simulink model "c00006M_harness"  (R2018a)
settings: Solver=FixedStepAuto  StartTime=0.0  StopTime=300  FixedStep=0.1  RelTol=1e-3
undefined symbols (not defined in the file): A1, hmax, PriorityTank, R1, R2, sigbuilder_block, TempThreshold
(part 15 of 66)

== system c00006M_harness/M205/Tank3 ==
  CT3 : Inport
  F3 : Inport  Port=2
  E3 : Inport  Port=3
  MR3 : Inport  Port=4
  T3 : Inport  Port=5
  EB3 : Inport  Port=6
  LL2 : Inport  Port=7
  Control : Subsystem
  Logical Operator : Logic  AllPortsSameDT=off  OutDataTypeStr=boolean
  MasterTankControl : Subsystem
  Memory : Memory
  Memory2 : Memory
  TankModel : Subsystem
  LL3 : Outport
  wires:
  TankModel/1(LiquidLevel) -> Memory/1, LL3/1
  Control/1(LiquidIn) -> Logical Operator/1
  Control/2(LiquidOut) -> TankModel/2(LiquidOut)
  Memory/1 -> MasterTankControl/2(LiquidTank3), Control/8(LiquidLevel)
  MR3/1 -> Control/3(ManualReference)
  CT3/1 -> Control/2(StartMaintenance), Control/1(ControlType)
  F3/1 -> Control/4(Fill)
  E3/1 -> Control/5(Empty)
  LL2/1 -> Memory2/1
  Memory2/1 -> MasterTankControl/1(LiquidTank2)
  EB3/1 -> Control/6(EmergencyButton)
  MasterTankControl/1(AllowTheTankFilling) -> Logical Operator/2
  Logical Operator/1 -> TankModel/1(LiquidIn)
  T3/1 -> Control/7(Temperature)

== system c00006M_harness/M206/Tank2 ==
  CT2 : Inport
  F2 : Inport  Port=2
  E2 : Inport  Port=3
  MR2 : Inport  Port=4
  T2 : Inport  Port=5
  EB2 : Inport  Port=6
  LL3 : Inport  Port=7
  Control : Subsystem
  Logical Operator : Logic  AllPortsSameDT=off  OutDataTypeStr=boolean
  MasterTankControl : Subsystem
  Memory : Memory
  Memory2 : Memory
  TankModel : Subsystem
  LL2 : Outport
  wires:
  TankModel/1(LiquidLevel) -> Memory/1, LL2/1
  Control/1(LiquidIn) -> Logical Operator/1
  Control/2(LiquidOut) -> TankModel/2(LiquidOut)
  Memory/1 -> Control/8(LiquidLevel), MasterTankControl/1(LiquidTank2)
  MR2/1 -> Control/3(ManualReference)
  CT2/1 -> Control/2(StartMaintenance), Control/1(ControlType)
  F2/1 -> Control/4(Fill)
  E2/1 -> Control/5(Empty)
  LL3/1 -> Memory2/1
  Memory2/1 -> MasterTankControl/2(LiquidTank3)
  EB2/1 -> Control/6(EmergencyButton)
  MasterTankControl/1(AllowTheTankFilling) -> Logical Operator/2
  Logical Operator/1 -> TankModel/1(LiquidIn)
  T2/1 -> Control/7(Temperature)

== system c00006M_harness/M206/Tank3 ==
  CT3 : Inport
  F3 : Inport  Port=2
  E3 : Inport  Port=3
  MR3 : Inport  Port=4
  T3 : Inport  Port=5
  EB3 : Inport  Port=6
  LL2 : Inport  Port=7
  Control : Subsystem
  Logical Operator : Logic  AllPortsSameDT=off  OutDataTypeStr=boolean
  MasterTankControl : Subsystem
  Memory : Memory
  Memory2 : Memory
  TankModel : Subsystem
  LL3 : Outport
  wires:
  TankModel/1(LiquidLevel) -> Memory/1, LL3/1
  Control/1(LiquidIn) -> Logical Operator/1
  Control/2(LiquidOut) -> TankModel/2(LiquidOut)
  Memory/1 -> MasterTankControl/2(LiquidTank3), Control/8(LiquidLevel)
  MR3/1 -> Control/3(ManualReference)
  CT3/1 -> Control/2(StartMaintenance), Control/1(ControlType)
  F3/1 -> Control/4(Fill)
  E3/1 -> Control/5(Empty)
  LL2/1 -> Memory2/1
  Memory2/1 -> MasterTankControl/1(LiquidTank2)
  EB3/1 -> Control/6(EmergencyButton)
  MasterTankControl/1(AllowTheTankFilling) -> Logical Operator/2
  Logical Operator/1 -> TankModel/1(LiquidIn)
  T3/1 -> Control/7(Temperature)

== system c00006M_harness/M207/Tank2 ==
  CT2 : Inport
  F2 : Inport  Port=2
  E2 : Inport  Port=3
  MR2 : Inport  Port=4
  T2 : Inport  Port=5
  EB2 : Inport  Port=6
  LL3 : Inport  Port=7
  Control : Subsystem
  Logical Operator : Logic  AllPortsSameDT=off  OutDataTypeStr=boolean
  MasterTankControl : Subsystem
  Memory : Memory
  Memory2 : Memory
  TankModel : Subsystem
  LL2 : Outport
  wires:
  TankModel/1(LiquidLevel) -> Memory/1, LL2/1
  Control/1(LiquidIn) -> Logical Operator/1
  Control/2(LiquidOut) -> TankModel/2(LiquidOut)
  Memory/1 -> Control/8(LiquidLevel), MasterTankControl/1(LiquidTank2)
  MR2/1 -> Control/3(ManualReference)
  CT2/1 -> Control/2(StartMaintenance), Control/1(ControlType)
  F2/1 -> Control/4(Fill)
  E2/1 -> Control/5(Empty)
  LL3/1 -> Memory2/1
  Memory2/1 -> MasterTankControl/2(LiquidTank3)
  EB2/1 -> Control/6(EmergencyButton)
  MasterTankControl/1(AllowTheTankFilling) -> Logical Operator/2
  Logical Operator/1 -> TankModel/1(LiquidIn)
  T2/1 -> Control/7(Temperature)

== system c00006M_harness/M207/Tank3 ==
  CT3 : Inport
  F3 : Inport  Port=2
  E3 : Inport  Port=3
  MR3 : Inport  Port=4
  T3 : Inport  Port=5
  EB3 : Inport  Port=6
  LL2 : Inport  Port=7
  Control : Subsystem
  Logical Operator : Logic  AllPortsSameDT=off  OutDataTypeStr=boolean
  MasterTankControl : Subsystem
  Memory : Memory
  Memory2 : Memory
  TankModel : Subsystem
  LL3 : Outport
  wires:
  TankModel/1(LiquidLevel) -> Memory/1, LL3/1
  Control/1(LiquidIn) -> Logical Operator/1
  Control/2(LiquidOut) -> TankModel/2(LiquidOut)
  Memory/1 -> MasterTankControl/2(LiquidTank3), Control/8(LiquidLevel)
  MR3/1 -> Control/3(ManualReference)
  CT3/1 -> Control/2(StartMaintenance), Control/1(ControlType)
  F3/1 -> Control/4(Fill)
  E3/1 -> Control/5(Empty)
  LL2/1 -> Memory2/1
  Memory2/1 -> MasterTankControl/1(LiquidTank2)
  EB3/1 -> Control/6(EmergencyButton)
  MasterTankControl/1(AllowTheTankFilling) -> Logical Operator/2
  Logical Operator/1 -> TankModel/1(LiquidIn)
  T3/1 -> Control/7(Temperature)

== system c00006M_harness/M208/Tank2 ==
  CT2 : Inport
  F2 : Inport  Port=2
  E2 : Inport  Port=3
  MR2 : Inport  Port=4
  T2 : Inport  Port=5
  EB2 : Inport  Port=6
  LL3 : Inport  Port=7
  Control : Subsystem
  Logical Operator : Logic  AllPortsSameDT=off  OutDataTypeStr=boolean
  MasterTankControl : Subsystem
  Memory : Memory
  Memory2 : Memory
  TankModel : Subsystem
  LL2 : Outport
  wires:
  TankModel/1(LiquidLevel) -> Memory/1, LL2/1
  Control/1(LiquidIn) -> Logical Operator/1
  Control/2(LiquidOut) -> TankModel/2(LiquidOut)
  Memory/1 -> Control/8(LiquidLevel), MasterTankControl/1(LiquidTank2)
  MR2/1 -> Control/3(ManualReference)
  CT2/1 -> Control/2(StartMaintenance), Control/1(ControlType)
  F2/1 -> Control/4(Fill)
  E2/1 -> Control/5(Empty)
  LL3/1 -> Memory2/1
  Memory2/1 -> MasterTankControl/2(LiquidTank3)
  EB2/1 -> Control/6(EmergencyButton)
  MasterTankControl/1(AllowTheTankFilling) -> Logical Operator/2
  Logical Operator/1 -> TankModel/1(LiquidIn)
  T2/1 -> Control/7(Temperature)

== system c00006M_harness/M208/Tank3 ==
  CT3 : Inport
  F3 : Inport  Port=2
  E3 : Inport  Port=3
  MR3 : Inport  Port=4
  T3 : Inport  Port=5
  EB3 : Inport  Port=6
  LL2 : Inport  Port=7
  Control : Subsystem
  Logical Operator : Logic  AllPortsSameDT=off  OutDataTypeStr=boolean
  MasterTankControl : Subsystem
  Memory : Memory
  Memory2 : Memory
  TankModel : Subsystem
  LL3 : Outport
  wires:
  TankModel/1(LiquidLevel) -> Memory/1, LL3/1
  Control/1(LiquidIn) -> Logical Operator/1
  Control/2(LiquidOut) -> TankModel/2(LiquidOut)
  Memory/1 -> MasterTankControl/2(LiquidTank3), Control/8(LiquidLevel)
  MR3/1 -> Control/3(ManualReference)
  CT3/1 -> Control/2(StartMaintenance), Control/1(ControlType)
  F3/1 -> Control/4(Fill)
  E3/1 -> Control/5(Empty)
  LL2/1 -> Memory2/1
  Memory2/1 -> MasterTankControl/1(LiquidTank2)
  EB3/1 -> Control/6(EmergencyButton)
  MasterTankControl/1(AllowTheTankFilling) -> Logical Operator/2
  Logical Operator/1 -> TankModel/1(LiquidIn)
  T3/1 -> Control/7(Temperature)

== system c00006M_harness/M209/Tank2 ==
  CT2 : Inport
  F2 : Inport  Port=2
  E2 : Inport  Port=3
  MR2 : Inport  Port=4
  T2 : Inport  Port=5
  EB2 : Inport  Port=6
  LL3 : Inport  Port=7
  Control : Subsystem
  Logical Operator : Logic  AllPortsSameDT=off  OutDataTypeStr=boolean
  MasterTankControl : Subsystem
  Memory : Memory
  Memory2 : Memory
  TankModel : Subsystem
  LL2 : Outport
  wires:
  TankModel/1(LiquidLevel) -> Memory/1, LL2/1
  Control/1(LiquidIn) -> Logical Operator/1
  Control/2(LiquidOut) -> TankModel/2(LiquidOut)
  Memory/1 -> Control/8(LiquidLevel), MasterTankControl/1(LiquidTank2)
  MR2/1 -> Control/3(ManualReference)
  CT2/1 -> Control/2(StartMaintenance), Control/1(ControlType)
  F2/1 -> Control/4(Fill)
  E2/1 -> Control/5(Empty)
  LL3/1 -> Memory2/1
  Memory2/1 -> MasterTankControl/2(LiquidTank3)
  EB2/1 -> Control/6(EmergencyButton)
  MasterTankControl/1(AllowTheTankFilling) -> Logical Operator/2
  Logical Operator/1 -> TankModel/1(LiquidIn)
  T2/1 -> Control/7(Temperature)

== system c00006M_harness/M209/Tank3 ==
  CT3 : Inport
  F3 : Inport  Port=2
  E3 : Inport  Port=3
  MR3 : Inport  Port=4
  T3 : Inport  Port=5
  EB3 : Inport  Port=6
  LL2 : Inport  Port=7
  Control : Subsystem
  Logical Operator : Logic  AllPortsSameDT=off  OutDataTypeStr=boolean
  MasterTankControl : Subsystem
  Memory : Memory
  Memory2 : Memory
  TankModel : Subsystem
  LL3 : Outport
  wires:
  TankModel/1(LiquidLevel) -> Memory/1, LL3/1
  Control/1(LiquidIn) -> Logical Operator/1
  Control/2(LiquidOut) -> TankModel/2(LiquidOut)
  Memory/1 -> MasterTankControl/2(LiquidTank3), Control/8(LiquidLevel)
  MR3/1 -> Control/3(ManualReference)
  CT3/1 -> Control/2(StartMaintenance), Control/1(ControlType)
  F3/1 -> Control/4(Fill)
  E3/1 -> Control/5(Empty)
  LL2/1 -> Memory2/1
  Memory2/1 -> MasterTankControl/1(LiquidTank2)
  EB3/1 -> Control/6(EmergencyButton)
  MasterTankControl/1(AllowTheTankFilling) -> Logical Operator/2
  Logical Operator/1 -> TankModel/1(LiquidIn)
  T3/1 -> Control/7(Temperature)

== system c00006M_harness/M210/Tank2 ==
  CT2 : Inport
  F2 : Inport  Port=2
  E2 : Inport  Port=3
  MR2 : Inport  Port=4
  T2 : Inport  Port=5
  EB2 : Inport  Port=6
  LL3 : Inport  Port=7
  Control : Subsystem
  Logical Operator : Logic  AllPortsSameDT=off  OutDataTypeStr=boolean
  MasterTankControl : Subsystem
  Memory : Memory
  Memory2 : Memory
  TankModel : Subsystem
  LL2 : Outport
  wires:
  TankModel/1(LiquidLevel) -> Memory/1, LL2/1
  Control/1(LiquidIn) -> Logical Operator/1
  Control/2(LiquidOut) -> TankModel/2(LiquidOut)
  Memory/1 -> Control/8(LiquidLevel), MasterTankControl/1(LiquidTank2)
  MR2/1 -> Control/3(ManualReference)
  CT2/1 -> Control/2(StartMaintenance), Control/1(ControlType)
  F2/1 -> Control/4(Fill)
  E2/1 -> Control/5(Empty)
  LL3/1 -> Memory2/1
  Memory2/1 -> MasterTankControl/2(LiquidTank3)
  EB2/1 -> Control/6(EmergencyButton)
  MasterTankControl/1(AllowTheTankFilling) -> Logical Operator/2
  Logical Operator/1 -> TankModel/1(LiquidIn)
  T2/1 -> Control/7(Temperature)

== system c00006M_harness/M210/Tank3 ==
  CT3 : Inport
  F3 : Inport  Port=2
  E3 : Inport  Port=3
  MR3 : Inport  Port=4
  T3 : Inport  Port=5
  EB3 : Inport  Port=6
  LL2 : Inport  Port=7
  Control : Subsystem
  Logical Operator : Logic  AllPortsSameDT=off  OutDataTypeStr=boolean
  MasterTankControl : Subsystem
  Memory : Memory
  Memory2 : Memory
  TankModel : Subsystem
  LL3 : Outport
  wires:
  TankModel/1(LiquidLevel) -> Memory/1, LL3/1
  Control/1(LiquidIn) -> Logical Operator/1
  Control/2(LiquidOut) -> TankModel/2(LiquidOut)
  Memory/1 -> MasterTankControl/2(LiquidTank3), Control/8(LiquidLevel)
  MR3/1 -> Control/3(ManualReference)
  CT3/1 -> Control/2(StartMaintenance), Control/1(ControlType)
  F3/1 -> Control/4(Fill)
  E3/1 -> Control/5(Empty)
  LL2/1 -> Memory2/1
  Memory2/1 -> MasterTankControl/1(LiquidTank2)
  EB3/1 -> Control/6(EmergencyButton)
  MasterTankControl/1(AllowTheTankFilling) -> Logical Operator/2
  Logical Operator/1 -> TankModel/1(LiquidIn)
  T3/1 -> Control/7(Temperature)

== system c00006M_harness/M211/Tank2 ==
  CT2 : Inport
  F2 : Inport  Port=2
  E2 : Inport  Port=3
  MR2 : Inport  Port=4
  T2 : Inport  Port=5
  EB2 : Inport  Port=6
  LL3 : Inport  Port=7
  Control : Subsystem
  Logical Operator : Logic  AllPortsSameDT=off  OutDataTypeStr=boolean
  MasterTankControl : Subsystem
  Memory : Memory
  Memory2 : Memory
  TankModel : Subsystem
  LL2 : Outport
  wires:
  TankModel/1(LiquidLevel) -> Memory/1, LL2/1
  Control/1(LiquidIn) -> Logical Operator/1
  Control/2(LiquidOut) -> TankModel/2(LiquidOut)
  Memory/1 -> Control/8(LiquidLevel), MasterTankControl/1(LiquidTank2)
  MR2/1 -> Control/3(ManualReference)
  CT2/1 -> Control/2(StartMaintenance), Control/1(ControlType)
  F2/1 -> Control/4(Fill)
  E2/1 -> Control/5(Empty)
  LL3/1 -> Memory2/1
  Memory2/1 -> MasterTankControl/2(LiquidTank3)
  EB2/1 -> Control/6(EmergencyButton)
  MasterTankControl/1(AllowTheTankFilling) -> Logical Operator/2
  Logical Operator/1 -> TankModel/1(LiquidIn)
  T2/1 -> Control/7(Temperature)

== system c00006M_harness/M211/Tank3 ==
  CT3 : Inport
  F3 : Inport  Port=2
  E3 : Inport  Port=3
  MR3 : Inport  Port=4
  T3 : Inport  Port=5
  EB3 : Inport  Port=6
  LL2 : Inport  Port=7
  Control : Subsystem
  Logical Operator : Logic  AllPortsSameDT=off  OutDataTypeStr=boolean
  MasterTankControl : Subsystem
  Memory : Memory
  Memory2 : Memory
  TankModel : Subsystem
  LL3 : Outport
  wires:
  TankModel/1(LiquidLevel) -> Memory/1, LL3/1
  Control/1(LiquidIn) -> Logical Operator/1
  Control/2(LiquidOut) -> TankModel/2(LiquidOut)
  Memory/1 -> MasterTankControl/2(LiquidTank3), Control/8(LiquidLevel)
  MR3/1 -> Control/3(ManualReference)
  CT3/1 -> Control/2(StartMaintenance), Control/1(ControlType)
  F3/1 -> Control/4(Fill)
  E3/1 -> Control/5(Empty)
  LL2/1 -> Memory2/1
  Memory2/1 -> MasterTankControl/1(LiquidTank2)
  EB3/1 -> Control/6(EmergencyButton)
  MasterTankControl/1(AllowTheTankFilling) -> Logical Operator/2
  Logical Operator/1 -> TankModel/1(LiquidIn)
  T3/1 -> Control/7(Temperature)

== system c00006M_harness/M212/Tank2 ==
  CT2 : Inport
  F2 : Inport  Port=2
  E2 : Inport  Port=3
  MR2 : Inport  Port=4
  T2 : Inport  Port=5
  EB2 : Inport  Port=6
  LL3 : Inport  Port=7
  Control : Subsystem
  Logical Operator : Logic  AllPortsSameDT=off  OutDataTypeStr=boolean
  MasterTankControl : Subsystem
  Memory : Memory
  Memory2 : Memory
  TankModel : Subsystem
  LL2 : Outport
  wires:
  TankModel/1(LiquidLevel) -> Memory/1, LL2/1
  Control/1(LiquidIn) -> Logical Operator/1
  Control/2(LiquidOut) -> TankModel/2(LiquidOut)
  Memory/1 -> Control/8(LiquidLevel), MasterTankControl/1(LiquidTank2)
  MR2/1 -> Control/3(ManualReference)
  CT2/1 -> Control/2(StartMaintenance), Control/1(ControlType)
  F2/1 -> Control/4(Fill)
  E2/1 -> Control/5(Empty)
  LL3/1 -> Memory2/1
  Memory2/1 -> MasterTankControl/2(LiquidTank3)
  EB2/1 -> Control/6(EmergencyButton)
  MasterTankControl/1(AllowTheTankFilling) -> Logical Operator/2
  Logical Operator/1 -> TankModel/1(LiquidIn)
  T2/1 -> Control/7(Temperature)

== system c00006M_harness/M212/Tank3 ==
  CT3 : Inport
  F3 : Inport  Port=2
  E3 : Inport  Port=3
  MR3 : Inport  Port=4
  T3 : Inport  Port=5
  EB3 : Inport  Port=6
  LL2 : Inport  Port=7
  Control : Subsystem
  Logical Operator : Logic  AllPortsSameDT=off  OutDataTypeStr=boolean
  MasterTankControl : Subsystem
  Memory : Memory
  Memory2 : Memory
  TankModel : Subsystem
  LL3 : Outport
  wires:
  TankModel/1(LiquidLevel) -> Memory/1, LL3/1
  Control/1(LiquidIn) -> Logical Operator/1
  Control/2(LiquidOut) -> TankModel/2(LiquidOut)
  Memory/1 -> MasterTankControl/2(LiquidTank3), Control/8(LiquidLevel)
  MR3/1 -> Control/3(ManualReference)
  CT3/1 -> Control/2(StartMaintenance), Control/1(ControlType)
  F3/1 -> Control/4(Fill)
  E3/1 -> Control/5(Empty)
  LL2/1 -> Memory2/1
  Memory2/1 -> MasterTankControl/1(LiquidTank2)
  EB3/1 -> Control/6(EmergencyButton)
  MasterTankControl/1(AllowTheTankFilling) -> Logical Operator/2
  Logical Operator/1 -> TankModel/1(LiquidIn)
  T3/1 -> Control/7(Temperature)

== system c00006M_harness/M213/Tank2 ==
  CT2 : Inport
  F2 : Inport  Port=2
  E2 : Inport  Port=3
  MR2 : Inport  Port=4
  T2 : Inport  Port=5
  EB2 : Inport  Port=6
  LL3 : Inport  Port=7
  Control : Subsystem
  Logical Operator : Logic  AllPortsSameDT=off  OutDataTypeStr=boolean
  MasterTankControl : Subsystem
  Memory : Memory
  Memory2 : Memory
  TankModel : Subsystem
  LL2 : Outport
  wires:
  TankModel/1(LiquidLevel) -> Memory/1, LL2/1
  Control/1(LiquidIn) -> Logical Operator/1
  Control/2(LiquidOut) -> TankModel/2(LiquidOut)
  Memory/1 -> Control/8(LiquidLevel), MasterTankControl/1(LiquidTank2)
  MR2/1 -> Control/3(ManualReference)
  CT2/1 -> Control/2(StartMaintenance), Control/1(ControlType)
  F2/1 -> Control/4(Fill)
  E2/1 -> Control/5(Empty)
  LL3/1 -> Memory2/1
  Memory2/1 -> MasterTankControl/2(LiquidTank3)
  EB2/1 -> Control/6(EmergencyButton)
  MasterTankControl/1(AllowTheTankFilling) -> Logical Operator/2
  Logical Operator/1 -> TankModel/1(LiquidIn)
  T2/1 -> Control/7(Temperature)

== system c00006M_harness/M213/Tank3 ==
  CT3 : Inport
  F3 : Inport  Port=2
  E3 : Inport  Port=3
  MR3 : Inport  Port=4
  T3 : Inport  Port=5
  EB3 : Inport  Port=6
  LL2 : Inport  Port=7
  Control : Subsystem
  Logical Operator : Logic  AllPortsSameDT=off  OutDataTypeStr=boolean
  MasterTankControl : Subsystem
  Memory : Memory
  Memory2 : Memory
  TankModel : Subsystem
  LL3 : Outport
  wires:
  TankModel/1(LiquidLevel) -> Memory/1, LL3/1
  Control/1(LiquidIn) -> Logical Operator/1
  Control/2(LiquidOut) -> TankModel/2(LiquidOut)
  Memory/1 -> MasterTankControl/2(LiquidTank3), Control/8(LiquidLevel)
  MR3/1 -> Control/3(ManualReference)
  CT3/1 -> Control/2(StartMaintenance), Control/1(ControlType)
  F3/1 -> Control/4(Fill)
  E3/1 -> Control/5(Empty)
  LL2/1 -> Memory2/1
  Memory2/1 -> MasterTankControl/1(LiquidTank2)
  EB3/1 -> Control/6(EmergencyButton)
  MasterTankControl/1(AllowTheTankFilling) -> Logical Operator/2
  Logical Operator/1 -> TankModel/1(LiquidIn)
  T3/1 -> Control/7(Temperature)

== system c00006M_harness/M214/Tank2 ==
  CT2 : Inport
  F2 : Inport  Port=2
  E2 : Inport  Port=3
  MR2 : Inport  Port=4
  T2 : Inport  Port=5
  EB2 : Inport  Port=6
  LL3 : Inport  Port=7
  Control : Subsystem
  Logical Operator : Logic  AllPortsSameDT=off  OutDataTypeStr=boolean
  MasterTankControl : Subsystem
  Memory : Memory
  Memory2 : Memory
  TankModel : Subsystem
  LL2 : Outport
  wires:
  TankModel/1(LiquidLevel) -> Memory/1, LL2/1
  Control/1(LiquidIn) -> Logical Operator/1
  Control/2(LiquidOut) -> TankModel/2(LiquidOut)
  Memory/1 -> Control/8(LiquidLevel), MasterTankControl/1(LiquidTank2)
  MR2/1 -> Control/3(ManualReference)
  CT2/1 -> Control/2(StartMaintenance), Control/1(ControlType)
  F2/1 -> Control/4(Fill)
  E2/1 -> Control/5(Empty)
  LL3/1 -> Memory2/1
  Memory2/1 -> MasterTankControl/2(LiquidTank3)
  EB2/1 -> Control/6(EmergencyButton)
  MasterTankControl/1(AllowTheTankFilling) -> Logical Operator/2
  Logical Operator/1 -> TankModel/1(LiquidIn)
  T2/1 -> Control/7(Temperature)

== system c00006M_harness/M214/Tank3 ==
  CT3 : Inport
  F3 : Inport  Port=2
  E3 : Inport  Port=3
  MR3 : Inport  Port=4
  T3 : Inport  Port=5
  EB3 : Inport  Port=6
  LL2 : Inport  Port=7
  Control : Subsystem
  Logical Operator : Logic  AllPortsSameDT=off  OutDataTypeStr=boolean
  MasterTankControl : Subsystem
  Memory : Memory
  Memory2 : Memory
  TankModel : Subsystem
  LL3 : Outport
  wires:
  TankModel/1(LiquidLevel) -> Memory/1, LL3/1
  Control/1(LiquidIn) -> Logical Operator/1
  Control/2(LiquidOut) -> TankModel/2(LiquidOut)
  Memory/1 -> MasterTankControl/2(LiquidTank3), Control/8(LiquidLevel)
  MR3/1 -> Control/3(ManualReference)
  CT3/1 -> Control/2(StartMaintenance), Control/1(ControlType)
  F3/1 -> Control/4(Fill)
  E3/1 -> Control/5(Empty)
  LL2/1 -> Memory2/1
  Memory2/1 -> MasterTankControl/1(LiquidTank2)
  EB3/1 -> Control/6(EmergencyButton)
  MasterTankControl/1(AllowTheTankFilling) -> Logical Operator/2
  Logical Operator/1 -> TankModel/1(LiquidIn)
  T3/1 -> Control/7(Temperature)

== system c00006M_harness/M215/Tank2 ==
  CT2 : Inport
  F2 : Inport  Port=2
  E2 : Inport  Port=3
  MR2 : Inport  Port=4
  T2 : Inport  Port=5
  EB2 : Inport  Port=6
  LL3 : Inport  Port=7
  Control : Subsystem
  Logical Operator : Logic  AllPortsSameDT=off  OutDataTypeStr=boolean
  MasterTankControl : Subsystem
  Memory : Memory
  Memory2 : Memory
  TankModel : Subsystem
  LL2 : Outport
  wires:
  TankModel/1(LiquidLevel) -> Memory/1, LL2/1
  Control/1(LiquidIn) -> Logical Operator/1
  Control/2(LiquidOut) -> TankModel/2(LiquidOut)
  Memory/1 -> Control/8(LiquidLevel), MasterTankControl/1(LiquidTank2)
  MR2/1 -> Control/3(ManualReference)
  CT2/1 -> Control/2(StartMaintenance), Control/1(ControlType)
  F2/1 -> Control/4(Fill)
  E2/1 -> Control/5(Empty)
  LL3/1 -> Memory2/1
  Memory2/1 -> MasterTankControl/2(LiquidTank3)
  EB2/1 -> Control/6(EmergencyButton)
  MasterTankControl/1(AllowTheTankFilling) -> Logical Operator/2
  Logical Operator/1 -> TankModel/1(LiquidIn)
  T2/1 -> Control/7(Temperature)

== system c00006M_harness/M215/Tank3 ==
  CT3 : Inport
  F3 : Inport  Port=2
  E3 : Inport  Port=3
  MR3 : Inport  Port=4
  T3 : Inport  Port=5
  EB3 : Inport  Port=6
  LL2 : Inport  Port=7
  Control : Subsystem
  Logical Operator : Logic  AllPortsSameDT=off  OutDataTypeStr=boolean
  MasterTankControl : Subsystem
  Memory : Memory
  Memory2 : Memory
  TankModel : Subsystem
  LL3 : Outport
  wires:
  TankModel/1(LiquidLevel) -> Memory/1, LL3/1
  Control/1(LiquidIn) -> Logical Operator/1
  Control/2(LiquidOut) -> TankModel/2(LiquidOut)
  Memory/1 -> MasterTankControl/2(LiquidTank3), Control/8(LiquidLevel)
  MR3/1 -> Control/3(ManualReference)
  CT3/1 -> Control/2(StartMaintenance), Control/1(ControlType)
  F3/1 -> Control/4(Fill)
  E3/1 -> Control/5(Empty)
  LL2/1 -> Memory2/1
  Memory2/1 -> MasterTankControl/1(LiquidTank2)
  EB3/1 -> Control/6(EmergencyButton)
  MasterTankControl/1(AllowTheTankFilling) -> Logical Operator/2
  Logical Operator/1 -> TankModel/1(LiquidIn)
  T3/1 -> Control/7(Temperature)

== system c00006M_harness/M216/Tank2 ==
  CT2 : Inport
  F2 : Inport  Port=2
  E2 : Inport  Port=3
  MR2 : Inport  Port=4
  T2 : Inport  Port=5
  EB2 : Inport  Port=6
  LL3 : Inport  Port=7
  Control : Subsystem
  Logical Operator : Logic  AllPortsSameDT=off  OutDataTypeStr=boolean
  MasterTankControl : Subsystem
  Memory : Memory
  Memory2 : Memory
  TankModel : Subsystem
  LL2 : Outport
  wires:
  TankModel/1(LiquidLevel) -> Memory/1, LL2/1
  Control/1(LiquidIn) -> Logical Operator/1
  Control/2(LiquidOut) -> TankModel/2(LiquidOut)
  Memory/1 -> Control/8(LiquidLevel), MasterTankControl/1(LiquidTank2)
  MR2/1 -> Control/3(ManualReference)
  CT2/1 -> Control/2(StartMaintenance), Control/1(ControlType)
  F2/1 -> Control/4(Fill)
  E2/1 -> Control/5(Empty)
  LL3/1 -> Memory2/1
  Memory2/1 -> MasterTankControl/2(LiquidTank3)
  EB2/1 -> Control/6(EmergencyButton)
  MasterTankControl/1(AllowTheTankFilling) -> Logical Operator/2
  Logical Operator/1 -> TankModel/1(LiquidIn)
  T2/1 -> Control/7(Temperature)

== system c00006M_harness/M216/Tank3 ==
  CT3 : Inport
  F3 : Inport  Port=2
  E3 : Inport  Port=3
  MR3 : Inport  Port=4
  T3 : Inport  Port=5
  EB3 : Inport  Port=6
  LL2 : Inport  Port=7
  Control : Subsystem
  Logical Operator : Logic  AllPortsSameDT=off  OutDataTypeStr=boolean
  MasterTankControl : Subsystem
  Memory : Memory
  Memory2 : Memory
  TankModel : Subsystem
  LL3 : Outport
  wires:
  TankModel/1(LiquidLevel) -> Memory/1, LL3/1
  Control/1(LiquidIn) -> Logical Operator/1
  Control/2(LiquidOut) -> TankModel/2(LiquidOut)
  Memory/1 -> MasterTankControl/2(LiquidTank3), Control/8(LiquidLevel)
  MR3/1 -> Control/3(ManualReference)
  CT3/1 -> Control/2(StartMaintenance), Control/1(ControlType)
  F3/1 -> Control/4(Fill)
  E3/1 -> Control/5(Empty)
  LL2/1 -> Memory2/1
  Memory2/1 -> MasterTankControl/1(LiquidTank2)
  EB3/1 -> Control/6(EmergencyButton)
  MasterTankControl/1(AllowTheTankFilling) -> Logical Operator/2
  Logical Operator/1 -> TankModel/1(LiquidIn)
  T3/1 -> Control/7(Temperature)

== system c00006M_harness/M217/Tank2 ==
  CT2 : Inport
  F2 : Inport  Port=2
  E2 : Inport  Port=3
  MR2 : Inport  Port=4
  T2 : Inport  Port=5
  EB2 : Inport  Port=6
  LL3 : Inport  Port=7
  Control : Subsystem
  Logical Operator : Logic  AllPortsSameDT=off  OutDataTypeStr=boolean
  MasterTankControl : Subsystem
  Memory : Memory
  Memory2 : Memory
  TankModel : Subsystem
  LL2 : Outport
  wires:
  TankModel/1(LiquidLevel) -> Memory/1, LL2/1
  Control/1(LiquidIn) -> Logical Operator/1
  Control/2(LiquidOut) -> TankModel/2(LiquidOut)
  Memory/1 -> Control/8(LiquidLevel), MasterTankControl/1(LiquidTank2)
  MR2/1 -> Control/3(ManualReference)
  CT2/1 -> Control/2(StartMaintenance), Control/1(ControlType)
  F2/1 -> Control/4(Fill)
  E2/1 -> Control/5(Empty)
  LL3/1 -> Memory2/1
  Memory2/1 -> MasterTankControl/2(LiquidTank3)
  EB2/1 -> Control/6(EmergencyButton)
  MasterTankControl/1(AllowTheTankFilling) -> Logical Operator/2
  Logical Operator/1 -> TankModel/1(LiquidIn)
  T2/1 -> Control/7(Temperature)

== system c00006M_harness/M217/Tank3 ==
  CT3 : Inport
  F3 : Inport  Port=2
  E3 : Inport  Port=3
  MR3 : Inport  Port=4
  T3 : Inport  Port=5
  EB3 : Inport  Port=6
  LL2 : Inport  Port=7
  Control : Subsystem
  Logical Operator : Logic  AllPortsSameDT=off  OutDataTypeStr=boolean
  MasterTankControl : Subsystem
  Memory : Memory
  Memory2 : Memory
  TankModel : Subsystem
  LL3 : Outport
  wires:
  TankModel/1(LiquidLevel) -> Memory/1, LL3/1
  Control/1(LiquidIn) -> Logical Operator/1
  Control/2(LiquidOut) -> TankModel/2(LiquidOut)
  Memory/1 -> MasterTankControl/2(LiquidTank3), Control/8(LiquidLevel)
  MR3/1 -> Control/3(ManualReference)
  CT3/1 -> Control/2(StartMaintenance), Control/1(ControlType)
  F3/1 -> Control/4(Fill)
  E3/1 -> Control/5(Empty)
  LL2/1 -> Memory2/1
  Memory2/1 -> MasterTankControl/1(LiquidTank2)
  EB3/1 -> Control/6(EmergencyButton)
  MasterTankControl/1(AllowTheTankFilling) -> Logical Operator/2
  Logical Operator/1 -> TankModel/1(LiquidIn)
  T3/1 -> Control/7(Temperature)

== system c00006M_harness/M218/Tank2 ==
  CT2 : Inport
  F2 : Inport  Port=2
  E2 : Inport  Port=3
  MR2 : Inport  Port=4
  T2 : Inport  Port=5
  EB2 : Inport  Port=6
  LL3 : Inport  Port=7
  Control : Subsystem
  Logical Operator : Logic  AllPortsSameDT=off  OutDataTypeStr=boolean
  MasterTankControl : Subsystem
  Memory : Memory
  Memory2 : Memory
  TankModel : Subsystem
  LL2 : Outport
  wires:
  TankModel/1(LiquidLevel) -> Memory/1, LL2/1
  Control/1(LiquidIn) -> Logical Operator/1
  Control/2(LiquidOut) -> TankModel/2(LiquidOut)
  Memory/1 -> Control/8(LiquidLevel), MasterTankControl/1(LiquidTank2)
  MR2/1 -> Control/3(ManualReference)
  CT2/1 -> Control/2(StartMaintenance), Control/1(ControlType)
  F2/1 -> Control/4(Fill)
  E2/1 -> Control/5(Empty)
  LL3/1 -> Memory2/1
  Memory2/1 -> MasterTankControl/2(LiquidTank3)
  EB2/1 -> Control/6(EmergencyButton)
  MasterTankControl/1(AllowTheTankFilling) -> Logical Operator/2
  Logical Operator/1 -> TankModel/1(LiquidIn)
  T2/1 -> Control/7(Temperature)

== system c00006M_harness/M218/Tank3 ==
  CT3 : Inport
  F3 : Inport  Port=2
  E3 : Inport  Port=3
  MR3 : Inport  Port=4
  T3 : Inport  Port=5
  EB3 : Inport  Port=6
  LL2 : Inport  Port=7
  Control : Subsystem
  Logical Operator : Logic  AllPortsSameDT=off  OutDataTypeStr=boolean
  MasterTankControl : Subsystem
  Memory : Memory
  Memory2 : Memory
  TankModel : Subsystem
  LL3 : Outport
  wires:
  TankModel/1(LiquidLevel) -> Memory/1, LL3/1
  Control/1(LiquidIn) -> Logical Operator/1
  Control/2(LiquidOut) -> TankModel/2(LiquidOut)
  Memory/1 -> MasterTankControl/2(LiquidTank3), Control/8(LiquidLevel)
  MR3/1 -> Control/3(ManualReference)
  CT3/1 -> Control/2(StartMaintenance), Control/1(ControlType)
  F3/1 -> Control/4(Fill)
  E3/1 -> Control/5(Empty)
  LL2/1 -> Memory2/1
  Memory2/1 -> MasterTankControl/1(LiquidTank2)
  EB3/1 -> Control/6(EmergencyButton)
  MasterTankControl/1(AllowTheTankFilling) -> Logical Operator/2
  Logical Operator/1 -> TankModel/1(LiquidIn)
  T3/1 -> Control/7(Temperature)

== system c00006M_harness/M219/Tank2 ==
  CT2 : Inport
  F2 : Inport  Port=2
  E2 : Inport  Port=3
  MR2 : Inport  Port=4
  T2 : Inport  Port=5
  EB2 : Inport  Port=6
  LL3 : Inport  Port=7
  Control : Subsystem
  Logical Operator : Logic  AllPortsSameDT=off  OutDataTypeStr=boolean
  MasterTankControl : Subsystem
  Memory : Memory
  Memory2 : Memory
  TankModel : Subsystem
  LL2 : Outport
  wires:
  TankModel/1(LiquidLevel) -> Memory/1, LL2/1
  Control/1(LiquidIn) -> Logical Operator/1
  Control/2(LiquidOut) -> TankModel/2(LiquidOut)
  Memory/1 -> Control/8(LiquidLevel), MasterTankControl/1(LiquidTank2)
  MR2/1 -> Control/3(ManualReference)
  CT2/1 -> Control/2(StartMaintenance), Control/1(ControlType)
  F2/1 -> Control/4(Fill)
  E2/1 -> Control/5(Empty)
  LL3/1 -> Memory2/1
  Memory2/1 -> MasterTankControl/2(LiquidTank3)
  EB2/1 -> Control/6(EmergencyButton)
  MasterTankControl/1(AllowTheTankFilling) -> Logical Operator/2
  Logical Operator/1 -> TankModel/1(LiquidIn)
  T2/1 -> Control/7(Temperature)

== system c00006M_harness/M219/Tank3 ==
  CT3 : Inport
  F3 : Inport  Port=2
  E3 : Inport  Port=3
  MR3 : Inport  Port=4
  T3 : Inport  Port=5
  EB3 : Inport  Port=6
  LL2 : Inport  Port=7
  Control : Subsystem
  Logical Operator : Logic  AllPortsSameDT=off  OutDataTypeStr=boolean
  MasterTankControl : Subsystem
  Memory : Memory
  Memory2 : Memory
  TankModel : Subsystem
  LL3 : Outport
  wires:
  TankModel/1(LiquidLevel) -> Memory/1, LL3/1
  Control/1(LiquidIn) -> Logical Operator/1
  Control/2(LiquidOut) -> TankModel/2(LiquidOut)
  Memory/1 -> MasterTankControl/2(LiquidTank3), Control/8(LiquidLevel)
  MR3/1 -> Control/3(ManualReference)
  CT3/1 -> Control/2(StartMaintenance), Control/1(ControlType)
  F3/1 -> Control/4(Fill)
  E3/1 -> Control/5(Empty)
  LL2/1 -> Memory2/1
  Memory2/1 -> MasterTankControl/1(LiquidTank2)
  EB3/1 -> Control/6(EmergencyButton)
  MasterTankControl/1(AllowTheTankFilling) -> Logical Operator/2
  Logical Operator/1 -> TankModel/1(LiquidIn)
  T3/1 -> Control/7(Temperature)

== system c00006M_harness/M220/Tank2 ==
  CT2 : Inport
  F2 : Inport  Port=2
  E2 : Inport  Port=3
  MR2 : Inport  Port=4
  T2 : Inport  Port=5
  EB2 : Inport  Port=6
  LL3 : Inport  Port=7
  Control : Subsystem
  Logical Operator : Logic  AllPortsSameDT=off  OutDataTypeStr=boolean
  MasterTankControl : Subsystem
  Memory : Memory
  Memory2 : Memory
  TankModel : Subsystem
  LL2 : Outport
  wires:
  TankModel/1(LiquidLevel) -> Memory/1, LL2/1
  Control/1(LiquidIn) -> Logical Operator/1
  Control/2(LiquidOut) -> TankModel/2(LiquidOut)
  Memory/1 -> Control/8(LiquidLevel), MasterTankControl/1(LiquidTank2)
  MR2/1 -> Control/3(ManualReference)
  CT2/1 -> Control/2(StartMaintenance), Control/1(ControlType)
  F2/1 -> Control/4(Fill)
  E2/1 -> Control/5(Empty)
  LL3/1 -> Memory2/1
  Memory2/1 -> MasterTankControl/2(LiquidTank3)
  EB2/1 -> Control/6(EmergencyButton)
  MasterTankControl/1(AllowTheTankFilling) -> Logical Operator/2
  Logical Operator/1 -> TankModel/1(LiquidIn)
  T2/1 -> Control/7(Temperature)

== system c00006M_harness/M220/Tank3 ==
  CT3 : Inport
  F3 : Inport  Port=2
  E3 : Inport  Port=3
  MR3 : Inport  Port=4
  T3 : Inport  Port=5
  EB3 : Inport  Port=6
  LL2 : Inport  Port=7
  Control : Subsystem
  Logical Operator : Logic  AllPortsSameDT=off  OutDataTypeStr=boolean
  MasterTankControl : Subsystem
  Memory : Memory
  Memory2 : Memory
  TankModel : Subsystem
  LL3 : Outport
  wires:
  TankModel/1(LiquidLevel) -> Memory/1, LL3/1
  Control/1(LiquidIn) -> Logical Operator/1
  Control/2(LiquidOut) -> TankModel/2(LiquidOut)
  Memory/1 -> MasterTankControl/2(LiquidTank3), Control/8(LiquidLevel)
  MR3/1 -> Control/3(ManualReference)
  CT3/1 -> Control/2(StartMaintenance), Control/1(ControlType)
  F3/1 -> Control/4(Fill)
  E3/1 -> Control/5(Empty)
  LL2/1 -> Memory2/1
  Memory2/1 -> MasterTankControl/1(LiquidTank2)
  EB3/1 -> Control/6(EmergencyButton)
  MasterTankControl/1(AllowTheTankFilling) -> Logical Operator/2
  Logical Operator/1 -> TankModel/1(LiquidIn)
  T3/1 -> Control/7(Temperature)

== system c00006M_harness/M221/Tank2 ==
  CT2 : Inport
  F2 : Inport  Port=2
  E2 : Inport  Port=3
  MR2 : Inport  Port=4
  T2 : Inport  Port=5
  EB2 : Inport  Port=6
  LL3 : Inport  Port=7
  Control : Subsystem
  Logical Operator : Logic  AllPortsSameDT=off  OutDataTypeStr=boolean
  MasterTankControl : Subsystem
  Memory : Memory
  Memory2 : Memory
  TankModel : Subsystem
  LL2 : Outport
  wires:
  TankModel/1(LiquidLevel) -> Memory/1, LL2/1
  Control/1(LiquidIn) -> Logical Operator/1
  Control/2(LiquidOut) -> TankModel/2(LiquidOut)
  Memory/1 -> Control/8(LiquidLevel), MasterTankControl/1(LiquidTank2)
  MR2/1 -> Control/3(ManualReference)
  CT2/1 -> Control/2(StartMaintenance), Control/1(ControlType)
  F2/1 -> Control/4(Fill)
  E2/1 -> Control/5(Empty)
  LL3/1 -> Memory2/1
  Memory2/1 -> MasterTankControl/2(LiquidTank3)
  EB2/1 -> Control/6(EmergencyButton)
  MasterTankControl/1(AllowTheTankFilling) -> Logical Operator/2
  Logical Operator/1 -> TankModel/1(LiquidIn)
  T2/1 -> Control/7(Temperature)

== system c00006M_harness/M221/Tank3 ==
  CT3 : Inport
  F3 : Inport  Port=2
  E3 : Inport  Port=3
  MR3 : Inport  Port=4
  T3 : Inport  Port=5
  EB3 : Inport  Port=6
  LL2 : Inport  Port=7
  Control : Subsystem
  Logical Operator : Logic  AllPortsSameDT=off  OutDataTypeStr=boolean
  MasterTankControl : Subsystem
  Memory : Memory
  Memory2 : Memory
  TankModel : Subsystem
  LL3 : Outport
  wires:
  TankModel/1(LiquidLevel) -> Memory/1, LL3/1
  Control/1(LiquidIn) -> Logical Operator/1
  Control/2(LiquidOut) -> TankModel/2(LiquidOut)
  Memory/1 -> MasterTankControl/2(LiquidTank3), Control/8(LiquidLevel)
  MR3/1 -> Control/3(ManualReference)
  CT3/1 -> Control/2(StartMaintenance), Control/1(ControlType)
  F3/1 -> Control/4(Fill)
  E3/1 -> Control/5(Empty)
  LL2/1 -> Memory2/1
  Memory2/1 -> MasterTankControl/1(LiquidTank2)
  EB3/1 -> Control/6(EmergencyButton)
  MasterTankControl/1(AllowTheTankFilling) -> Logical Operator/2
  Logical Operator/1 -> TankModel/1(LiquidIn)
  T3/1 -> Control/7(Temperature)

== system c00006M_harness/M222/Tank2 ==
  CT2 : Inport
  F2 : Inport  Port=2
  E2 : Inport  Port=3
  MR2 : Inport  Port=4
  T2 : Inport  Port=5
  EB2 : Inport  Port=6
  LL3 : Inport  Port=7
  Control : Subsystem
  Logical Operator : Logic  AllPortsSameDT=off  OutDataTypeStr=boolean
  MasterTankControl : Subsystem
  Memory : Memory
  Memory2 : Memory
  TankModel : Subsystem
  LL2 : Outport
  wires:
  TankModel/1(LiquidLevel) -> Memory/1, LL2/1
  Control/1(LiquidIn) -> Logical Operator/1
  Control/2(LiquidOut) -> TankModel/2(LiquidOut)
  Memory/1 -> Control/8(LiquidLevel), MasterTankControl/1(LiquidTank2)
  MR2/1 -> Control/3(ManualReference)
  CT2/1 -> Control/2(StartMaintenance), Control/1(ControlType)
  F2/1 -> Control/4(Fill)
  E2/1 -> Control/5(Empty)
  LL3/1 -> Memory2/1
  Memory2/1 -> MasterTankControl/2(LiquidTank3)
  EB2/1 -> Control/6(EmergencyButton)
  MasterTankControl/1(AllowTheTankFilling) -> Logical Operator/2
  Logical Operator/1 -> TankModel/1(LiquidIn)
  T2/1 -> Control/7(Temperature)

== system c00006M_harness/M222/Tank3 ==
  CT3 : Inport
  F3 : Inport  Port=2
  E3 : Inport  Port=3
  MR3 : Inport  Port=4
  T3 : Inport  Port=5
  EB3 : Inport  Port=6
  LL2 : Inport  Port=7
  Control : Subsystem
  Logical Operator : Logic  AllPortsSameDT=off  OutDataTypeStr=boolean
  MasterTankControl : Subsystem
  Memory : Memory
  Memory2 : Memory
  TankModel : Subsystem
  LL3 : Outport
  wires:
  TankModel/1(LiquidLevel) -> Memory/1, LL3/1
  Control/1(LiquidIn) -> Logical Operator/1
  Control/2(LiquidOut) -> TankModel/2(LiquidOut)
  Memory/1 -> MasterTankControl/2(LiquidTank3), Control/8(LiquidLevel)
  MR3/1 -> Control/3(ManualReference)
  CT3/1 -> Control/2(StartMaintenance), Control/1(ControlType)
  F3/1 -> Control/4(Fill)
  E3/1 -> Control/5(Empty)
  LL2/1 -> Memory2/1
  Memory2/1 -> MasterTankControl/1(LiquidTank2)
  EB3/1 -> Control/6(EmergencyButton)
  MasterTankControl/1(AllowTheTankFilling) -> Logical Operator/2
  Logical Operator/1 -> TankModel/1(LiquidIn)
  T3/1 -> Control/7(Temperature)

== system c00006M_harness/M223/Tank2 ==
  CT2 : Inport
  F2 : Inport  Port=2
  E2 : Inport  Port=3
  MR2 : Inport  Port=4
  T2 : Inport  Port=5
  EB2 : Inport  Port=6
  LL3 : Inport  Port=7
  Control : Subsystem
  Logical Operator : Logic  AllPortsSameDT=off  OutDataTypeStr=boolean
  MasterTankControl : Subsystem
  Memory : Memory
  Memory2 : Memory
  TankModel : Subsystem
  LL2 : Outport
  wires:
  TankModel/1(LiquidLevel) -> Memory/1, LL2/1
  Control/1(LiquidIn) -> Logical Operator/1
  Control/2(LiquidOut) -> TankModel/2(LiquidOut)
  Memory/1 -> Control/8(LiquidLevel), MasterTankControl/1(LiquidTank2)
  MR2/1 -> Control/3(ManualReference)
  CT2/1 -> Control/2(StartMaintenance), Control/1(ControlType)
  F2/1 -> Control/4(Fill)
  E2/1 -> Control/5(Empty)
  LL3/1 -> Memory2/1
  Memory2/1 -> MasterTankControl/2(LiquidTank3)
  EB2/1 -> Control/6(EmergencyButton)
  MasterTankControl/1(AllowTheTankFilling) -> Logical Operator/2
  Logical Operator/1 -> TankModel/1(LiquidIn)
  T2/1 -> Control/7(Temperature)

== system c00006M_harness/M223/Tank3 ==
  CT3 : Inport
  F3 : Inport  Port=2
  E3 : Inport  Port=3
  MR3 : Inport  Port=4
  T3 : Inport  Port=5
  EB3 : Inport  Port=6
  LL2 : Inport  Port=7
  Control : Subsystem
  Logical Operator : Logic  AllPortsSameDT=off  OutDataTypeStr=boolean
  MasterTankControl : Subsystem
  Memory : Memory
  Memory2 : Memory
  TankModel : Subsystem
  LL3 : Outport
  wires:
  TankModel/1(LiquidLevel) -> Memory/1, LL3/1
  Control/1(LiquidIn) -> Logical Operator/1
  Control/2(LiquidOut) -> TankModel/2(LiquidOut)
  Memory/1 -> MasterTankControl/2(LiquidTank3), Control/8(LiquidLevel)
  MR3/1 -> Control/3(ManualReference)
  CT3/1 -> Control/2(StartMaintenance), Control/1(ControlType)
  F3/1 -> Control/4(Fill)
  E3/1 -> Control/5(Empty)
  LL2/1 -> Memory2/1
  Memory2/1 -> MasterTankControl/1(LiquidTank2)
  EB3/1 -> Control/6(EmergencyButton)
  MasterTankControl/1(AllowTheTankFilling) -> Logical Operator/2
  Logical Operator/1 -> TankModel/1(LiquidIn)
  T3/1 -> Control/7(Temperature)

== system c00006M_harness/M224/Tank2 ==
  CT2 : Inport
  F2 : Inport  Port=2
  E2 : Inport  Port=3
  MR2 : Inport  Port=4
  T2 : Inport  Port=5
  EB2 : Inport  Port=6
  LL3 : Inport  Port=7
  Control : Subsystem
  Logical Operator : Logic  AllPortsSameDT=off  OutDataTypeStr=boolean
  MasterTankControl : Subsystem
  Memory : Memory
  Memory2 : Memory
  TankModel : Subsystem
  LL2 : Outport
  wires:
  TankModel/1(LiquidLevel) -> Memory/1, LL2/1
  Control/1(LiquidIn) -> Logical Operator/1
  Control/2(LiquidOut) -> TankModel/2(LiquidOut)
  Memory/1 -> Control/8(LiquidLevel), MasterTankControl/1(LiquidTank2)
  MR2/1 -> Control/3(ManualReference)
  CT2/1 -> Control/2(StartMaintenance), Control/1(ControlType)
  F2/1 -> Control/4(Fill)
  E2/1 -> Control/5(Empty)
  LL3/1 -> Memory2/1
  Memory2/1 -> MasterTankControl/2(LiquidTank3)
  EB2/1 -> Control/6(EmergencyButton)
  MasterTankControl/1(AllowTheTankFilling) -> Logical Operator/2
  Logical Operator/1 -> TankModel/1(LiquidIn)
  T2/1 -> Control/7(Temperature)

== system c00006M_harness/M224/Tank3 ==
  CT3 : Inport
  F3 : Inport  Port=2
  E3 : Inport  Port=3
  MR3 : Inport  Port=4
  T3 : Inport  Port=5
  EB3 : Inport  Port=6
  LL2 : Inport  Port=7
  Control : Subsystem
  Logical Operator : Logic  AllPortsSameDT=off  OutDataTypeStr=boolean
  MasterTankControl : Subsystem
  Memory : Memory
  Memory2 : Memory
  TankModel : Subsystem
  LL3 : Outport
  wires:
  TankModel/1(LiquidLevel) -> Memory/1, LL3/1
  Control/1(LiquidIn) -> Logical Operator/1
  Control/2(LiquidOut) -> TankModel/2(LiquidOut)
  Memory/1 -> MasterTankControl/2(LiquidTank3), Control/8(LiquidLevel)
  MR3/1 -> Control/3(ManualReference)
  CT3/1 -> Control/2(StartMaintenance), Control/1(ControlType)
  F3/1 -> Control/4(Fill)
  E3/1 -> Control/5(Empty)
  LL2/1 -> Memory2/1
  Memory2/1 -> MasterTankControl/1(LiquidTank2)
  EB3/1 -> Control/6(EmergencyButton)
  MasterTankControl/1(AllowTheTankFilling) -> Logical Operator/2
  Logical Operator/1 -> TankModel/1(LiquidIn)
  T3/1 -> Control/7(Temperature)

== system c00006M_harness/M225/Tank2 ==
  CT2 : Inport
  F2 : Inport  Port=2
  E2 : Inport  Port=3
  MR2 : Inport  Port=4
  T2 : Inport  Port=5
  EB2 : Inport  Port=6
  LL3 : Inport  Port=7
  Control : Subsystem
  Logical Operator : Logic  AllPortsSameDT=off  OutDataTypeStr=boolean
  MasterTankControl : Subsystem
  Memory : Memory
  Memory2 : Memory
  TankModel : Subsystem
  LL2 : Outport
  wires:
  TankModel/1(LiquidLevel) -> Memory/1, LL2/1
  Control/1(LiquidIn) -> Logical Operator/1
  Control/2(LiquidOut) -> TankModel/2(LiquidOut)
  Memory/1 -> Control/8(LiquidLevel), MasterTankControl/1(LiquidTank2)
  MR2/1 -> Control/3(ManualReference)
  CT2/1 -> Control/2(StartMaintenance), Control/1(ControlType)
  F2/1 -> Control/4(Fill)
  E2/1 -> Control/5(Empty)
  LL3/1 -> Memory2/1
  Memory2/1 -> MasterTankControl/2(LiquidTank3)
  EB2/1 -> Control/6(EmergencyButton)
  MasterTankControl/1(AllowTheTankFilling) -> Logical Operator/2
  Logical Operator/1 -> TankModel/1(LiquidIn)
  T2/1 -> Control/7(Temperature)

== system c00006M_harness/M225/Tank3 ==
  CT3 : Inport
  F3 : Inport  Port=2
  E3 : Inport  Port=3
  MR3 : Inport  Port=4
  T3 : Inport  Port=5
  EB3 : Inport  Port=6
  LL2 : Inport  Port=7
  Control : Subsystem
  Logical Operator : Logic  AllPortsSameDT=off  OutDataTypeStr=boolean
  MasterTankControl : Subsystem
  Memory : Memory
  Memory2 : Memory
  TankModel : Subsystem
  LL3 : Outport
  wires:
  TankModel/1(LiquidLevel) -> Memory/1, LL3/1
  Control/1(LiquidIn) -> Logical Operator/1
  Control/2(LiquidOut) -> TankModel/2(LiquidOut)
  Memory/1 -> MasterTankControl/2(LiquidTank3), Control/8(LiquidLevel)
  MR3/1 -> Control/3(ManualReference)
  CT3/1 -> Control/2(StartMaintenance), Control/1(ControlType)
  F3/1 -> Control/4(Fill)
  E3/1 -> Control/5(Empty)
  LL2/1 -> Memory2/1
  Memory2/1 -> MasterTankControl/1(LiquidTank2)
  EB3/1 -> Control/6(EmergencyButton)
  MasterTankControl/1(AllowTheTankFilling) -> Logical Operator/2
  Logical Operator/1 -> TankModel/1(LiquidIn)
  T3/1 -> Control/7(Temperature)

== system c00006M_harness/M226/Tank2 ==
  CT2 : Inport
  F2 : Inport  Port=2
  E2 : Inport  Port=3
  MR2 : Inport  Port=4
  T2 : Inport  Port=5
  EB2 : Inport  Port=6
  LL3 : Inport  Port=7
  Control : Subsystem
  Logical Operator : Logic  AllPortsSameDT=off  OutDataTypeStr=boolean
  MasterTankControl : Subsystem
  Memory : Memory
  Memory2 : Memory
  TankModel : Subsystem
  LL2 : Outport
  wires:
  TankModel/1(LiquidLevel) -> Memory/1, LL2/1
  Control/1(LiquidIn) -> Logical Operator/1
  Control/2(LiquidOut) -> TankModel/2(LiquidOut)
  Memory/1 -> Control/8(LiquidLevel), MasterTankControl/1(LiquidTank2)
  MR2/1 -> Control/3(ManualReference)
  CT2/1 -> Control/2(StartMaintenance), Control/1(ControlType)
  F2/1 -> Control/4(Fill)
  E2/1 -> Control/5(Empty)
  LL3/1 -> Memory2/1
  Memory2/1 -> MasterTankControl/2(LiquidTank3)
  EB2/1 -> Control/6(EmergencyButton)
  MasterTankControl/1(AllowTheTankFilling) -> Logical Operator/2
  Logical Operator/1 -> TankModel/1(LiquidIn)
  T2/1 -> Control/7(Temperature)

== system c00006M_harness/M226/Tank3 ==
  CT3 : Inport
  F3 : Inport  Port=2
  E3 : Inport  Port=3
  MR3 : Inport  Port=4
  T3 : Inport  Port=5
  EB3 : Inport  Port=6
  LL2 : Inport  Port=7
  Control : Subsystem
  Logical Operator : Logic  Operator=OR  AllPortsSameDT=off  OutDataTypeStr=boolean
  MasterTankControl : Subsystem
  Memory : Memory
  Memory2 : Memory
  TankModel : Subsystem
  LL3 : Outport
  wires:
  TankModel/1(LiquidLevel) -> Memory/1, LL3/1
  Control/1(LiquidIn) -> Logical Operator/1
  Control/2(LiquidOut) -> TankModel/2(LiquidOut)
  Memory/1 -> MasterTankControl/2(LiquidTank3), Control/8(LiquidLevel)
  MR3/1 -> Control/3(ManualReference)
  CT3/1 -> Control/2(StartMaintenance), Control/1(ControlType)
  F3/1 -> Control/4(Fill)
  E3/1 -> Control/5(Empty)
  LL2/1 -> Memory2/1
  Memory2/1 -> MasterTankControl/1(LiquidTank2)
  EB3/1 -> Control/6(EmergencyButton)
  MasterTankControl/1(AllowTheTankFilling) -> Logical Operator/2
  Logical Operator/1 -> TankModel/1(LiquidIn)
  T3/1 -> Control/7(Temperature)

== system c00006M_harness/M227/Tank2 ==
  CT2 : Inport
  F2 : Inport  Port=2
  E2 : Inport  Port=3
  MR2 : Inport  Port=4
  T2 : Inport  Port=5
  EB2 : Inport  Port=6
  LL3 : Inport  Port=7
  Control : Subsystem
  Logical Operator : Logic  AllPortsSameDT=off  OutDataTypeStr=boolean
  MasterTankControl : Subsystem
  Memory : Memory
  Memory2 : Memory
  TankModel : Subsystem
  LL2 : Outport
  wires:
  TankModel/1(LiquidLevel) -> Memory/1, LL2/1
  Control/1(LiquidIn) -> Logical Operator/1
  Control/2(LiquidOut) -> TankModel/2(LiquidOut)
  Memory/1 -> Control/8(LiquidLevel), MasterTankControl/1(LiquidTank2)
  MR2/1 -> Control/3(ManualReference)
  CT2/1 -> Control/2(StartMaintenance), Control/1(ControlType)
  F2/1 -> Control/4(Fill)
  E2/1 -> Control/5(Empty)
  LL3/1 -> Memory2/1
  Memory2/1 -> MasterTankControl/2(LiquidTank3)
  EB2/1 -> Control/6(EmergencyButton)
  MasterTankControl/1(AllowTheTankFilling) -> Logical Operator/2
  Logical Operator/1 -> TankModel/1(LiquidIn)
  T2/1 -> Control/7(Temperature)

== system c00006M_harness/M227/Tank3 ==
  CT3 : Inport
  F3 : Inport  Port=2
  E3 : Inport  Port=3
  MR3 : Inport  Port=4
  T3 : Inport  Port=5
  EB3 : Inport  Port=6
  LL2 : Inport  Port=7
  Control : Subsystem
  Logical Operator : Logic  AllPortsSameDT=off  OutDataTypeStr=boolean
  MasterTankControl : Subsystem
  Memory : Memory
  Memory2 : Memory
  TankModel : Subsystem
  LL3 : Outport
  wires:
  TankModel/1(LiquidLevel) -> Memory/1, LL3/1
  Control/1(LiquidIn) -> Logical Operator/1
  Control/2(LiquidOut) -> TankModel/2(LiquidOut)
  Memory/1 -> MasterTankControl/2(LiquidTank3), Control/8(LiquidLevel)
  MR3/1 -> Control/3(ManualReference)
  CT3/1 -> Control/2(StartMaintenance), Control/1(ControlType)
  F3/1 -> Control/4(Fill)
  E3/1 -> Control/5(Empty)
  LL2/1 -> Memory2/1
  Memory2/1 -> MasterTankControl/1(LiquidTank2)
  EB3/1 -> Control/6(EmergencyButton)
  MasterTankControl/1(AllowTheTankFilling) -> Logical Operator/2
  Logical Operator/1 -> TankModel/1(LiquidIn)
  T3/1 -> Control/7(Temperature)

== system c00006M_harness/M228/Tank2 ==
  CT2 : Inport
  F2 : Inport  Port=2
  E2 : Inport  Port=3
  MR2 : Inport  Port=4
  T2 : Inport  Port=5
  EB2 : Inport  Port=6
  LL3 : Inport  Port=7
  Control : Subsystem
  Logical Operator : Logic  AllPortsSameDT=off  OutDataTypeStr=boolean
  MasterTankControl : Subsystem
  Memory : Memory
  Memory2 : Memory
  TankModel : Subsystem
  LL2 : Outport
  wires:
  TankModel/1(LiquidLevel) -> Memory/1, LL2/1
  Control/1(LiquidIn) -> Logical Operator/1
  Control/2(LiquidOut) -> TankModel/2(LiquidOut)
  Memory/1 -> Control/8(LiquidLevel), MasterTankControl/1(LiquidTank2)
  MR2/1 -> Control/3(ManualReference)
  CT2/1 -> Control/2(StartMaintenance), Control/1(ControlType)
  F2/1 -> Control/4(Fill)
  E2/1 -> Control/5(Empty)
  LL3/1 -> Memory2/1
  Memory2/1 -> MasterTankControl/2(LiquidTank3)
  EB2/1 -> Control/6(EmergencyButton)
  MasterTankControl/1(AllowTheTankFilling) -> Logical Operator/2
  Logical Operator/1 -> TankModel/1(LiquidIn)
  T2/1 -> Control/7(Temperature)

== system c00006M_harness/M228/Tank3 ==
  CT3 : Inport
  F3 : Inport  Port=2
  E3 : Inport  Port=3
  MR3 : Inport  Port=4
  T3 : Inport  Port=5
  EB3 : Inport  Port=6
  LL2 : Inport  Port=7
  Control : Subsystem
  Logical Operator : Logic  AllPortsSameDT=off  OutDataTypeStr=boolean
  MasterTankControl : Subsystem
  Memory : Memory
  Memory2 : Memory
  TankModel : Subsystem
  LL3 : Outport
  wires:
  TankModel/1(LiquidLevel) -> Memory/1, LL3/1
  Control/1(LiquidIn) -> Logical Operator/1
  Control/2(LiquidOut) -> TankModel/2(LiquidOut)
  Memory/1 -> MasterTankControl/2(LiquidTank3), Control/8(LiquidLevel)
  MR3/1 -> Control/3(ManualReference)
  CT3/1 -> Control/2(StartMaintenance), Control/1(ControlType)
  F3/1 -> Control/4(Fill)
  E3/1 -> Control/5(Empty)
  LL2/1 -> Memory2/1
  Memory2/1 -> MasterTankControl/1(LiquidTank2)
  EB3/1 -> Control/6(EmergencyButton)
  MasterTankControl/1(AllowTheTankFilling) -> Logical Operator/2
  Logical Operator/1 -> TankModel/1(LiquidIn)
  T3/1 -> Control/7(Temperature)

== system c00006M_harness/M229/Tank2 ==
  CT2 : Inport
  F2 : Inport  Port=2
  E2 : Inport  Port=3
  MR2 : Inport  Port=4
  T2 : Inport  Port=5
  EB2 : Inport  Port=6
  LL3 : Inport  Port=7
  Control : Subsystem
  Logical Operator : Logic  AllPortsSameDT=off  OutDataTypeStr=boolean
  MasterTankControl : Subsystem
  Memory : Memory
  Memory2 : Memory
  TankModel : Subsystem
  LL2 : Outport
  wires:
  TankModel/1(LiquidLevel) -> Memory/1, LL2/1
  Control/1(LiquidIn) -> Logical Operator/1
  Control/2(LiquidOut) -> TankModel/2(LiquidOut)
  Memory/1 -> Control/8(LiquidLevel), MasterTankControl/1(LiquidTank2)
  MR2/1 -> Control/3(ManualReference)
  CT2/1 -> Control/2(StartMaintenance), Control/1(ControlType)
  F2/1 -> Control/4(Fill)
  E2/1 -> Control/5(Empty)
  LL3/1 -> Memory2/1
  Memory2/1 -> MasterTankControl/2(LiquidTank3)
  EB2/1 -> Control/6(EmergencyButton)
  MasterTankControl/1(AllowTheTankFilling) -> Logical Operator/2
  Logical Operator/1 -> TankModel/1(LiquidIn)
  T2/1 -> Control/7(Temperature)
